simulink library "ltd"  (Simulink 8.1)
settings: Solver=ode1  StartTime=0.0  StopTime=Inf  FixedStep=0.001  RelTol=1e-3
PostLoadFcn:
  | , if any(exist('dsrtsu_mdlpostloadfcn', 'file') == [2, 3, 6]), try dsrtsu_mdlpostloadfcn('Execute', bdroot); catch fprintf('Error in PostLoadFcn (dsrtsu_mdlpostloadfcn) for model "%s":\n %s\n', bdroot, lasterr); end, end,
undefined symbols (not defined in the file or in its folder): C_TICK_TIME_S, FALSE, KACC_ACCDecelMaintainTimer_ms, TRUE
libraries: simulink x1, hcu_lib x1
settings Model: DSRTSU_INTERNAL_RTI_VER=450  DSRTSU_INTERNAL_RTI_TYPE=rti1401  RTICANMMDATA=struct('GeneralSetupData',struct('modelroot','D:\ELN150201_TAIWAN\trunk\AdasDragon\software\sw_development\arch\app\acc','generalsettings',struct('filesettings',struct('destfolder',struct('Name','RTICANMM_FILES','Check',1),'buildfolder',struct('Name','.','Check',1),'AbsDestfolder',struct('Name','D:\ELN150201_TAIWAN\trunk\AdasDragon\software\sw_development\arch\app\acc\RTICANMM_FILES'),'AbsBuildfolder',struct('Name','D:\ELN150201_TAIWAN\trunk\AdasDragon\software\sw_development\arch\app\acc'))),'options',struct('addpaths',1,'rmpaths',1,'addtrcexclusion',logical(1),'cannavigator',struct('checkmonitoring',0),'show_usrtrc',0,'use_usrtrc',0),'advanced',struct('options',[1 1 1 1 1 1 1 1 1 1 1 1 1 1 1 1 1 1 1 1 1 1 1 1 1 1 1 1 1 1 1 1 1 1 1 1 1 1 1 1 1 1 1 1 1 1 1 1 1 1 1 1 1 1 1 1 1 1 1 1 1 1 1 1 1 1 1 1 1 1 1 1 1 1 1 1 1 1 1 1 1 1 1 1 1 1 1 1 1 1 1 1 1 1 1 1 1 1 1 1]),'MPSetup',{{}},'modelname','ltd','block','ltd'))  DSRTSU_INTERNAL_RTIFPGA=40  Creator=AT015555  LastModifiedBy=AT015555

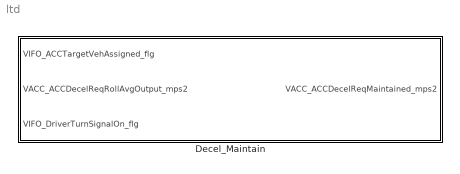
== system ltd ==
  Decel_Maintain : Subsystem

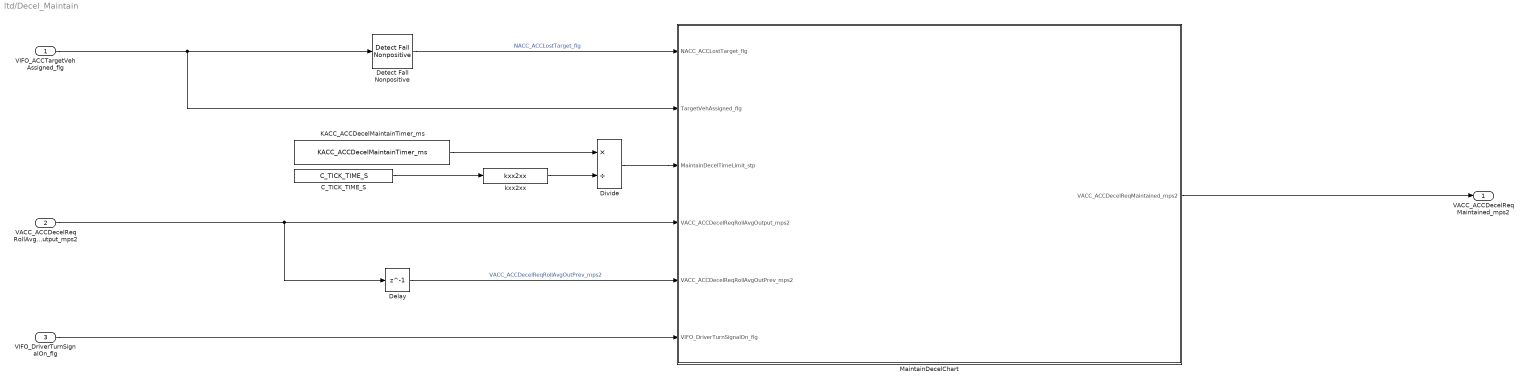
== system ltd/Decel_Maintain ==
  VIFO_ACCTargetVehAssigned_flg : Inport
  VACC_ACCDecelReqRollAvgOutput_mps2 : Inport  Port=2
  VIFO_DriverTurnSignalOn_flg : Inport  Port=3
  C_TICK_TIME_S : Constant  Value=C_TICK_TIME_S
  Delay : Delay  DelayLength=1  InitialCondition=0
  Detect Fall Nonpositive : simulink/Logic and Bit Operations/Detect Fall Nonpositive  vinit=0  InputProcessing=Inherited  OutDataTypeStr=boolean
  Divide : Product  Inputs=*/
  KACC_ACCDecelMaintainTimer_ms : Constant  Value=KACC_ACCDecelMaintainTimer_ms
  MaintainDecelChart : Stateflow chart  TreatAsAtomicUnit=on
  kxx2xx : hcu_lib/kxx2xx
  VACC_ACCDecelReqMaintained_mps2 : Outport
  wires:
  VIFO_ACCTargetVehAssigned_flg/1 -> MaintainDecelChart/2(TargetVehAssigned_flg), Detect Fall Nonpositive/1
  C_TICK_TIME_S/1 -> kxx2xx/1
  Divide/1 -> MaintainDecelChart/3(MaintainDecelTimeLimit_stp)
  kxx2xx/1 -> Divide/2
  KACC_ACCDecelMaintainTimer_ms/1 -> Divide/1
  VACC_ACCDecelReqRollAvgOutput_mps2/1 -> Delay/1, MaintainDecelChart/4(VACC_ACCDecelReqRollAvgOutput_mps2)
  Detect Fall Nonpositive/1 -> MaintainDecelChart/1(NACC_ACCLostTarget_flg)  "NACC_ACCLostTarget_flg"
  Delay/1 -> MaintainDecelChart/5(VACC_ACCDecelReqRollAvgOutPrev_mps2)  "VACC_ACCDecelReqRollAvgOutPrev_mps2"
  MaintainDecelChart/1(VACC_ACCDecelReqMaintained_mps2) -> VACC_ACCDecelReqMaintained_mps2/1
  VIFO_DriverTurnSignalOn_flg/1 -> MaintainDecelChart/6(VIFO_DriverTurnSignalOn_flg)

== stateflow chart Decel_Maintain/MaintainDecelChart ==
  state DIRECT_BRAKE
    du:
    VACC_ACCDecelReqMaintained_mps2 = VACC_ACCDecelReqRollAvgOutput_mps2;
  state MAINTAIN_LAST_DECEL
    en:
    MaintainDecelTimeLocal_stp = 0;
    du:
    MaintainDecelTimeLocal_stp=MaintainDecelTimeLocal_stp+1;
    ex:
    VACC_ACCDecelReqMaintained_mps2 = VACC_ACCDecelReqRollAvgOutput_mps2;
  state GET_LAST_DECEL
    en:
    VACC_ACCDecelReqMaintained_mps2 = VACC_ACCDecelReqRollAvgOutPrev_mps2;
  (default) -> DIRECT_BRAKE
  (junction 16) -> DIRECT_BRAKE : [MaintainDecelTimeLocal_stp>MaintainDecelTimeLimit_stp...
      | ||TargetVehAssigned_flg==TRUE]
  MAINTAIN_LAST_DECEL -> (junction 16)
  DIRECT_BRAKE -> (junction 17)
  GET_LAST_DECEL -> MAINTAIN_LAST_DECEL
  (junction 17) -> GET_LAST_DECEL : [NACC_ACCLostTarget_flg==TRUE...
      | &&VIFO_DriverTurnSignalOn_flg==FALSE]
  data: VACC_ACCDecelReqMaintained_mps2 output single; NACC_ACCLostTarget_flg input boolean; TargetVehAssigned_flg input boolean; MaintainDecelTimeLimit_stp input single; VACC_ACCDecelReqRollAvgOutput_mps2 input single; VACC_ACCDecelReqRollAvgOutPrev_mps2 input double; FALSE parameter double; TRUE parameter double; MaintainDecelTimeLocal_stp local single; VIFO_DriverTurnSignalOn_flg input double
